simulink library "srolib"  (Simulink 6.0)
settings: Solver=ode45  SolverMode=SingleTasking  StartTime=0.0  StopTime=10.0  RelTol=1e-3
undefined symbols (not defined in the file or in its folder): SignalConstrMask
settings Model: Creator=pascal  LastModifiedBy=pascal
settings DataIOCC: SignalLoggingName=logsOut
settings OptimizationCC: BooleanDataType=off
settings DebuggingCC: CheckExecutionContextPreStartOutputMsg=on  CheckExecutionContextRuntimeOutputMsg=on  SolverPrmCheckMsg=none
settings HardwareCC: TargetUnknown=on
settings ModelReferenceCC: UpdateModelReferenceTargets=IfOutOfDate
settings SFSimCC: SFSimApplyToAllLibs=on  SFSimBuildMode=Incremental

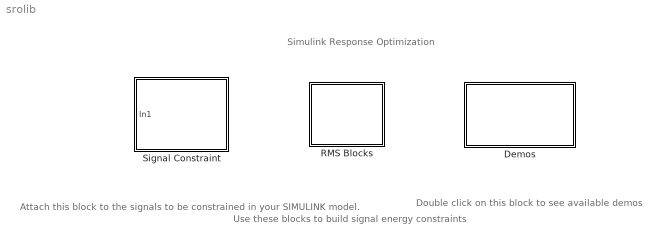
== system srolib ==
  note: Attach this block to
      | the signals to be constrained
      | in your SIMULINK model.
  note: Simulink Response Optimization
  note: Double click on this block
      | to see available demos
  note: Use these blocks to
      | build signal energy
      | constraints
  Demos : Subsystem  PropExecContextAcrossSSBoundary=on
      mask Display: disp('Response\nOptimization\nDemos')
  RMS Blocks : Subsystem  PropExecContextAcrossSSBoundary=on
      mask Display: disp('RMS\nBlocks')
  Signal Constraint : Subsystem  LoadFcn=SignalConstrMask('load',gcb)  PropExecContextAcrossSSBoundary=on  mask(Signal Constraint){DialogPosition=[0.1 0.25 0.45 0.31], SaveIn=workspace, SaveAs=, LogID=SRO_DataLog_1, Ylim=}
      mask prompts: DialogPosition "Dialog position"; SaveIn "Save constraint in"; SaveAs "Save constraint as"; LogID "Data Logging ID"; Ylim "Y axis limits"
      mask init:
      | % Apply logID to data logging port
      | b = find_system(gcb,'FollowLinks','on','LookUnderMasks','all','BlockType','SignalConversion');
      | h = get_param(b{1},'PortHandles');
      | set(h.Outport,'DataLoggingNameMode','custom',...
      | 	'DataLoggingName',LogID)
      settings: CopyFcn=SignalConstrMask('copy',gcb)  DeleteFcn=SignalConstrMask('delete',gcb)  UndoDeleteFcn=SignalConstrMask('undelete',gcb)  ModelCloseFcn=SignalConstrMask('modelclose',gcb)  PreSaveFcn=SignalConstrMask('save',gcb)  NameChangeFcn=SignalConstrMask('namechange',gcb)  OpenFcn=SignalConstrMask('open',gcb)  CloseFcn=SignalConstrMask('close',gcb)
      mask StyleString: edit,popup(workspace|MAT file),edit,edit,edit
      mask Display: plot([0:10],[-.5 1.5 .6 1.3 .8 1.1 .95 1.02 .99 1 1])

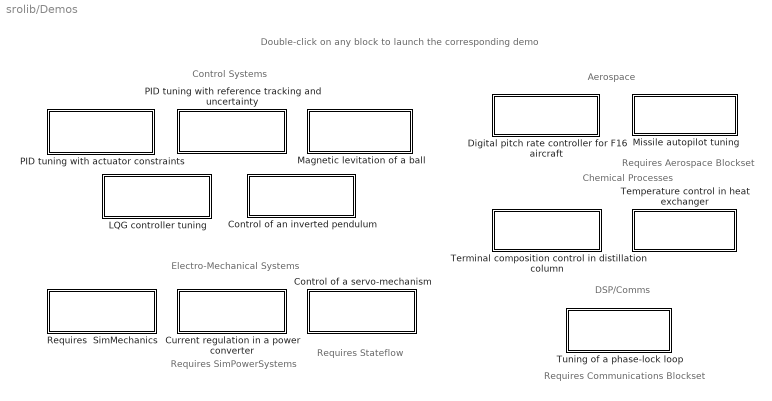
== system srolib/Demos ==
  note: Double-click on any block to launch the corresponding demo
  note: Control Systems
  note: Aerospace
  note: Chemical Processes
  note: DSP/Comms
  note: Electro-Mechanical Systems
  note: Requires
      | SimPowerSystems
  note: Requires
      | Stateflow
  note: Requires Communications
      | Blockset
  note: Requires Aerospace
      | Blockset
  Control of a servo-mechanism : Subsystem  PropExecContextAcrossSSBoundary=on  mask{A=}
      mask prompts: A "Nedded to invoke correct OpenFcn from Browser:"
      settings: OpenFcn=open_system('servo_demo')
      mask Display: disp('Servomechanism')
  Control of an inverted pendulum : Subsystem  PropExecContextAcrossSSBoundary=on  mask{A=}
      mask prompts: A "Nedded to invoke correct OpenFcn from Browser:"
      settings: OpenFcn=open_system('pendulum_demo')
      mask Display: disp('Inverted Pendulum')
  Current regulation in a power converter : Subsystem  PropExecContextAcrossSSBoundary=on  mask{A=}
      mask prompts: A "Nedded to invoke correct OpenFcn from Browser:"
      settings: OpenFcn=open_system('power_demo')
      mask Display: disp('Power Converter')
  Digital pitch rate controller for F16 aircraft : Subsystem  PropExecContextAcrossSSBoundary=on  mask{A=}
      mask prompts: A "Nedded to invoke correct OpenFcn from Browser:"
      settings: OpenFcn=open_system('pitchrate_demo')
      mask Display: disp('Pitch Rate Control')
  LQG controller tuning : Subsystem  PropExecContextAcrossSSBoundary=on  mask{A=}
      mask prompts: A "Nedded to invoke correct OpenFcn from Browser:"
      settings: OpenFcn=open_system('lqg_demo')
      mask Display: disp('LQG Controller')
  Magnetic levitation of a ball : Subsystem  PropExecContextAcrossSSBoundary=on  mask{A=}
      mask prompts: A "Nedded to invoke correct OpenFcn from Browser:"
      settings: OpenFcn=open_system('maglev_demo')
      mask Display: disp('Magnetic Levitation')
  Missile autopilot tuning : Subsystem  PropExecContextAcrossSSBoundary=on  mask{A=}
      mask prompts: A "Nedded to invoke correct OpenFcn from Browser:"
      settings: OpenFcn=open_system('missile_demo')
      mask Display: disp('Missile Autopilot')
  PID tuning with actuator constraints : Subsystem  PropExecContextAcrossSSBoundary=on  mask{A=}
      mask prompts: A "Nedded to invoke correct OpenFcn from Browser:"
      settings: OpenFcn=open_system('pidtune_demo')
      mask Display: disp('PID Tuning 1')
  PID tuning with reference tracking and uncertainty : Subsystem  PropExecContextAcrossSSBoundary=on  mask{A=}
      mask prompts: A "Nedded to invoke correct OpenFcn from Browser:"
      settings: OpenFcn=open_system('pidtrack_demo')
      mask Display: disp('PID Tuning 2')
  Requires  SimMechanics : Subsystem  PropExecContextAcrossSSBoundary=on  mask{A=}
      mask prompts: A "Nedded to invoke correct OpenFcn from Browser:"
      settings: OpenFcn=open_system('stewart_demo')
      mask Display: disp('Stewart Platform')
  Temperature control in heat exchanger : Subsystem  PropExecContextAcrossSSBoundary=on  mask{A=}
      mask prompts: A "Nedded to invoke correct OpenFcn from Browser:"
      settings: OpenFcn=open_system('heatex_demo')
      mask Display: disp('Heat Exchanger')
  Terminal composition control in distillation column : Subsystem  PropExecContextAcrossSSBoundary=on  mask{A=}
      mask prompts: A "Nedded to invoke correct OpenFcn from Browser:"
      settings: OpenFcn=open_system('distillation_demo')
      mask Display: disp('Distillation Column')
  Tuning of a phase-lock loop : Subsystem  PropExecContextAcrossSSBoundary=on  mask{A=}
      mask prompts: A "Nedded to invoke correct OpenFcn from Browser:"
      settings: OpenFcn=open_system('phaselock_demo')
      mask Display: disp('Phase Lock Loop')

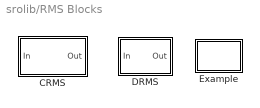
== system srolib/RMS Blocks ==
  CRMS : Subsystem  PropExecContextAcrossSSBoundary=on
      mask Type: Continuous RMS Value Block
      mask Description: Computes the cumulative root mean squared value of the input signal. The output is continuous.
      mask Display: disp('Continuous\nRMS');
  DRMS : Subsystem  PropExecContextAcrossSSBoundary=on  mask(Discrete RMS Value Block){Ts=1}
      mask prompts: Ts "Sampling Interval (s) :"
      mask help: Computes the cumulative root mean squared value of the sampled input signal. The output is discrete.
      mask Display: disp('Discrete\nRMS')
  Example : Subsystem  PropExecContextAcrossSSBoundary=on
      settings: OpenFcn=rmsdemo
      mask Type: DEMO
      mask Display: disp('DEMO')

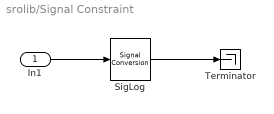
== system srolib/Signal Constraint ==
  In1 : Inport  LatchInput=off
  SigLog : SignalConversion  ConversionOutput=Contiguous copy  OverrideOpt=on
  Terminator : Terminator
  wires:
  In1/1 -> SigLog/1
  SigLog/1 -> Terminator/1

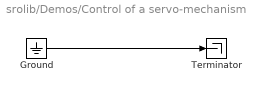
== system srolib/Demos/Control of a servo-mechanism ==
  Ground : Ground
  Terminator : Terminator
  wires:
  Ground/1 -> Terminator/1

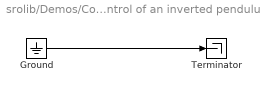
== system srolib/Demos/Control of an inverted pendulum ==
  Ground : Ground
  Terminator : Terminator
  wires:
  Ground/1 -> Terminator/1

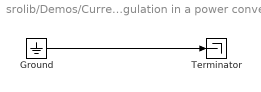
== system srolib/Demos/Current regulation in a power converter ==
  Ground : Ground
  Terminator : Terminator
  wires:
  Ground/1 -> Terminator/1

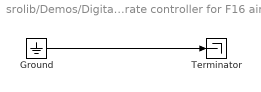
== system srolib/Demos/Digital pitch rate controller for F16 aircraft ==
  Ground : Ground
  Terminator : Terminator
  wires:
  Ground/1 -> Terminator/1

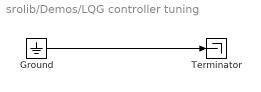
== system srolib/Demos/LQG controller tuning ==
  Ground : Ground
  Terminator : Terminator
  wires:
  Ground/1 -> Terminator/1

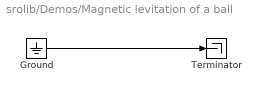
== system srolib/Demos/Magnetic levitation of a ball ==
  Ground : Ground
  Terminator : Terminator
  wires:
  Ground/1 -> Terminator/1

== system srolib/Demos/Missile autopilot tuning ==
  Ground : Ground
  Terminator : Terminator
  wires:
  Ground/1 -> Terminator/1

== system srolib/Demos/PID tuning with actuator constraints ==
  Ground : Ground
  Terminator : Terminator
  wires:
  Ground/1 -> Terminator/1

== system srolib/Demos/PID tuning with reference tracking and uncertainty ==
  Ground : Ground
  Terminator : Terminator
  wires:
  Ground/1 -> Terminator/1

== system srolib/Demos/Requires  SimMechanics ==

== system srolib/Demos/Temperature control in heat exchanger ==
  Ground : Ground
  Terminator : Terminator
  wires:
  Ground/1 -> Terminator/1

== system srolib/Demos/Terminal composition control in distillation column ==
  Ground : Ground
  Terminator : Terminator
  wires:
  Ground/1 -> Terminator/1

== system srolib/Demos/Tuning of a phase-lock loop ==
  Ground : Ground
  Terminator : Terminator
  wires:
  Ground/1 -> Terminator/1

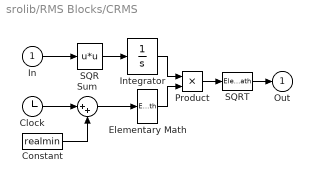
== system srolib/RMS Blocks/CRMS ==
  In : Inport  LatchInput=off
  Clock : Clock
      settings: Decimation=10
  Constant : Constant  Value=realmin
  Elementary Math : ElementaryMath  Operator=reciprocal
  Integrator : Integrator  LimitOutput=on  LowerSaturationLimit=0
  Product : Product  SaturateOnIntegerOverflow=on  InputSameDT=on
  SQR : Fcn  Expr=u*u
  SQRT : ElementaryMath  Operator=sqrt
  Sum : Sum  Inputs=|++
  Out : Outport  InitialOutput=0
  wires:
  In/1 -> SQR/1
  SQR/1 -> Integrator/1
  Integrator/1 -> Product/1
  Sum/1 -> Elementary Math/1
  Elementary Math/1 -> Product/2
  SQRT/1 -> Out/1
  Product/1 -> SQRT/1
  Constant/1 -> Sum/2
  Clock/1 -> Sum/1

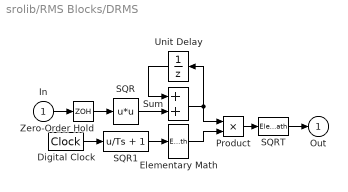
== system srolib/RMS Blocks/DRMS ==
  In : Inport  LatchInput=off
  Digital Clock : DigitalClock  SampleTime=Ts
  Elementary Math : ElementaryMath  Operator=reciprocal
  Product : Product  SaturateOnIntegerOverflow=on  InputSameDT=on
  SQR : Fcn  Expr=u*u
  SQR1 : Fcn  Expr=u/Ts + 1
  SQRT : ElementaryMath  Operator=sqrt
  Sum : Sum  SaturateOnIntegerOverflow=on  InputSameDT=on
  Unit Delay : UnitDelay  Orientation=left  SampleTime=Ts
  Zero-Order Hold : ZeroOrderHold  SampleTime=Ts
  Out : Outport  InitialOutput=0
  wires:
  SQR1/1 -> Elementary Math/1
  Digital Clock/1 -> SQR1/1
  SQRT/1 -> Out/1
  Product/1 -> SQRT/1
  Elementary Math/1 -> Product/2
  Unit Delay/1 -> Sum/1
  Sum/1 -> Unit Delay/1, Product/1
  SQR/1 -> Sum/2
  Zero-Order Hold/1 -> SQR/1
  In/1 -> Zero-Order Hold/1

== system srolib/RMS Blocks/Example ==
